simulink model "CoETS_TrqCalc"  (R2018a)
settings: configuration reference "cs_ert" (kept outside this file)
values from neighbouring files (symbols this model uses):
  DCSOVRDSENGPRT_SY : value not decoded    [CoETS_TrqCalc.sldd]
  ENGPRT_OVRDS_DCS : value not decoded    [CoETS_TrqCalc.sldd]
  PTPRTOVRDSSPDGOV_SY : value not decoded    [CoETS_TrqCalc.sldd]
  SPDGOV_OVRDS_PTPRT : value not decoded    [CoETS_TrqCalc.sldd]
settings Model: DataDictionary=CoETS_TrqCalc.sldd  Creator=zhoutinglin  LastModifiedBy=zhoutinglin

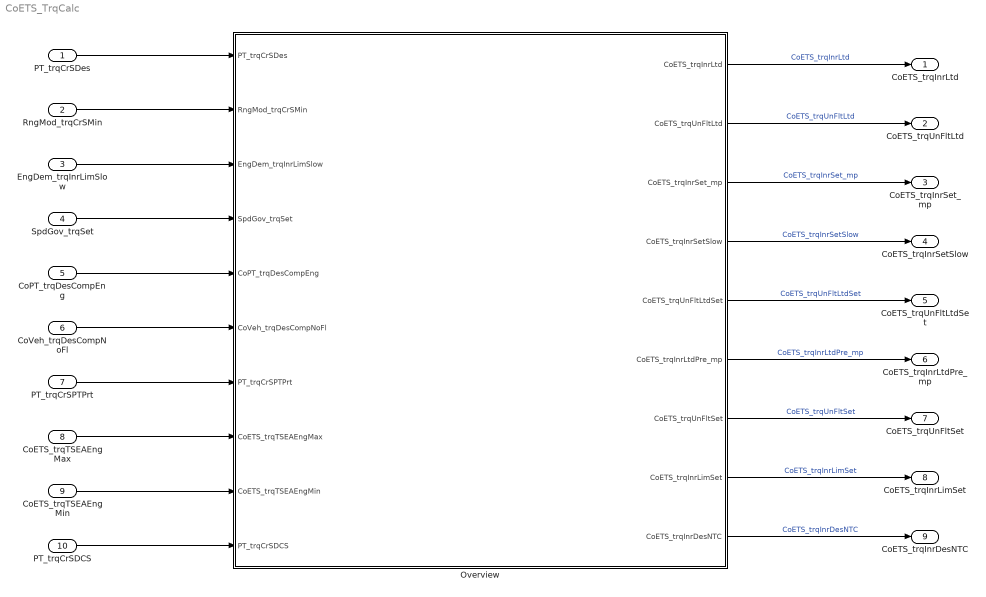
== system CoETS_TrqCalc ==
  PT_trqCrSDes : Inport  Description=application parameter for lead torque order to engine for rail pressure control（crankshaft torque）  OutMin=-3000  OutMax=3000  OutDataTypeStr=Torq  Unit=Nm  PortDimensions=[1 1]
  RngMod_trqCrSMin : Inport  Description=filtered setpoint torque of SpdGov  Port=2  OutMin=-3276.8  OutMax=3276.7  OutDataTypeStr=Torq  Unit=Nm  PortDimensions=[1 1]
  EngDem_trqInrLimSlow : Inport  Description=status speed control SpdGov  Port=3  OutMin=-3276.8  OutMax=3276.7  OutDataTypeStr=Torq  PortDimensions=[1 1]
  SpdGov_trqSet : Inport  Description=Resulting limiting torque (inner engine torque)  Port=4  OutMin=-3000  OutMax=3000  OutDataTypeStr=Torq  Unit=Nm  PortDimensions=[1 1]
  CoPT_trqDesCompEng : Inport  Description=inner engine limted lead torque  Port=5  OutMin=-3276  OutMax=3276  OutDataTypeStr=Torq  Unit=Nm  PortDimensions=[1 1]
  CoVeh_trqDesCompNoFl : Inport  Description=lead torque of SpdGov on the air path  Port=6  OutMin=-3000  OutMax=3000  OutDataTypeStr=Torq  Unit=Nm  PortDimensions=[1 1]
  PT_trqCrSPTPrt : Inport  Description=application parameter for lead torque order to engine（crankshaft torque）  Port=7  OutMin=-3000  OutMax=3000  OutDataTypeStr=Torq  Unit=Nm  PortDimensions=[1 1]
  CoETS_trqTSEAEngMax : Inport  Description=Application parameter for requested propulsion torque to engine(crankshaft torque)  Port=8  OutMin=-3276  OutMax=3276  OutDataTypeStr=Torq  Unit=Nm  PortDimensions=[1 1]
  CoETS_trqTSEAEngMin : Inport  Description=minimal crankshaft torque  Port=9  OutMin=-3276  OutMax=3276  OutDataTypeStr=Torq  Unit=Nm  PortDimensions=[1 1]
  PT_trqCrSDCS : Inport  Description=inner engine limted torque for Slow Path  Port=10  OutMin=-3000  OutMax=3000  OutDataTypeStr=Torq  Unit=Nm  PortDimensions=[1 1]
  Overview : Subsystem
  CoETS_trqInrLtd : Outport
  CoETS_trqUnFltLtd : Outport  Port=2
  CoETS_trqInrSet_mp : Outport  Port=3
  CoETS_trqInrSetSlow : Outport  Port=4
  CoETS_trqUnFltLtdSet : Outport  Port=5
  CoETS_trqInrLtdPre_mp : Outport  Port=6
  CoETS_trqUnFltSet : Outport  Port=7
  CoETS_trqInrLimSet : Outport  Port=8
  CoETS_trqInrDesNTC : Outport  Port=9
  wires:
  PT_trqCrSDes/1 -> Overview/1(PT_trqCrSDes)
  RngMod_trqCrSMin/1 -> Overview/2(RngMod_trqCrSMin)
  EngDem_trqInrLimSlow/1 -> Overview/3(EngDem_trqInrLimSlow)
  SpdGov_trqSet/1 -> Overview/4(SpdGov_trqSet)
  CoPT_trqDesCompEng/1 -> Overview/5(CoPT_trqDesCompEng)
  CoVeh_trqDesCompNoFl/1 -> Overview/6(CoVeh_trqDesCompNoFl)
  PT_trqCrSPTPrt/1 -> Overview/7(PT_trqCrSPTPrt)
  CoETS_trqTSEAEngMax/1 -> Overview/8(CoETS_trqTSEAEngMax)
  CoETS_trqTSEAEngMin/1 -> Overview/9(CoETS_trqTSEAEngMin)
  PT_trqCrSDCS/1 -> Overview/10(PT_trqCrSDCS)
  Overview/1(CoETS_trqInrLtd) -> CoETS_trqInrLtd/1  "CoETS_trqInrLtd"
  Overview/2(CoETS_trqUnFltLtd) -> CoETS_trqUnFltLtd/1  "CoETS_trqUnFltLtd"
  Overview/3(CoETS_trqInrSet_mp) -> CoETS_trqInrSet_mp/1  "CoETS_trqInrSet_mp"
  Overview/4(CoETS_trqInrSetSlow) -> CoETS_trqInrSetSlow/1  "CoETS_trqInrSetSlow"
  Overview/5(CoETS_trqUnFltLtdSet) -> CoETS_trqUnFltLtdSet/1  "CoETS_trqUnFltLtdSet"
  Overview/6(CoETS_trqInrLtdPre_mp) -> CoETS_trqInrLtdPre_mp/1  "CoETS_trqInrLtdPre_mp"
  Overview/7(CoETS_trqUnFltSet) -> CoETS_trqUnFltSet/1  "CoETS_trqUnFltSet"
  Overview/8(CoETS_trqInrLimSet) -> CoETS_trqInrLimSet/1  "CoETS_trqInrLimSet"
  Overview/9(CoETS_trqInrDesNTC) -> CoETS_trqInrDesNTC/1  "CoETS_trqInrDesNTC"

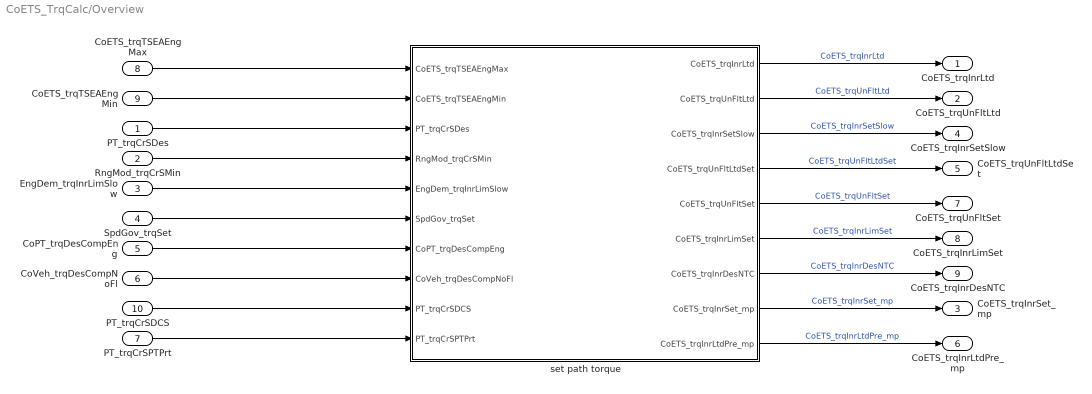
== system CoETS_TrqCalc/Overview ==
  PT_trqCrSDes : Inport  Tag=Nm  Description=Application parameter for requested propulsion torque to engine(crankshaft torque)  OutMin=-3000  OutMax=3000
  RngMod_trqCrSMin : Inport  Tag=Nm  Description=minimal crankshaft torque  Port=2  OutMin=-3276.8  OutMax=3276.7
  EngDem_trqInrLimSlow : Inport  Tag=Nm  Description=inner engine limted torque for Slow Path  Port=3  OutMin=-3276.8  OutMax=3276.7
  SpdGov_trqSet : Inport  Tag=Nm  Description=Set point torque of SpdGov on the fuel path  Port=4  OutMin=-3000  OutMax=3000
  CoPT_trqDesCompEng : Inport  Tag=Nm  Description=Application parameter for engine torque desired for compensation  Port=5  OutMin=-3276  OutMax=3276
  CoVeh_trqDesCompNoFl : Inport  Tag=Nm  Description=compensation torque with the shares,which not slur by the drive behaviour filter  Port=6  OutMin=-3000  OutMax=3000
  PT_trqCrSPTPrt : Inport  Tag=Nm  Description=Application parameter for powertrain protection train protection torque(crankshaft torque)  Port=7  OutMin=-3000  OutMax=3000
  CoETS_trqTSEAEngMax : Inport  Tag=Nm  Description=torque request to engine intervention decrement(Max)  Port=8  OutMin=-3276  OutMax=3276
  CoETS_trqTSEAEngMin : Inport  Tag=Nm  Description=torque request to engine intervention increment(Min)  Port=9  OutMin=-3276  OutMax=3276
  PT_trqCrSDCS : Inport  Tag=Nm  Description=crankshaft torque for request decrcment  Port=10  OutMin=-3000  OutMax=3000
  set path torque : Subsystem
  CoETS_trqInrLtd : Outport  Tag=Nm  Description=inner torque set value after limitation, before AS  OutMin=-3000  OutMax=3000
  CoETS_trqUnFltLtd : Outport  Tag=Nm  Description=Limited idle speed governor torque  Port=2  OutMin=-3276  OutMax=3276
  CoETS_trqInrSet_mp : Outport  Tag=Nm  Description=Intermediate inner torque for the set path without filteration  Port=3  OutMin=-3276  OutMax=3276
  CoETS_trqInrSetSlow : Outport  Tag=Nm  Description=Filtered inner torque ( positive torque) desired value (standard signal path) generated out of CoPT_trqDesEng  Port=4  OutMin=-3276  OutMax=3276
  CoETS_trqUnFltLtdSet : Outport  Tag=Nm  Description=Compensation torque of the accessories  Port=5  OutMin=-3276  OutMax=3276
  CoETS_trqInrLtdPre_mp : Outport  Tag=Nm  Description=inner set torque after limitation, before active surge damper  Port=6  OutMin=-3276  OutMax=3276
  CoETS_trqUnFltSet : Outport  Tag=Nm  Description="Compensation torque of \"loss torque compensation\" to bypass filter influences on the set path which is partly compensated"  Port=7  OutMin=-3276  OutMax=3276
  CoETS_trqInrLimSet : Outport  Tag=Nm  Description=Limitation torque without the part of the speed governor  Port=8  OutMin=-3000  OutMax=3000
  CoETS_trqInrDesNTC : Outport  Tag=Nm  Description=Additional desired engine friction Nm  Port=9  OutMin=-3276  OutMax=3276
  wires:
  set path torque/2(CoETS_trqUnFltLtd) -> CoETS_trqUnFltLtd/1  "CoETS_trqUnFltLtd"
  set path torque/4(CoETS_trqUnFltLtdSet) -> CoETS_trqUnFltLtdSet/1  "CoETS_trqUnFltLtdSet"
  SpdGov_trqSet/1 -> set path torque/6(SpdGov_trqSet)
  set path torque/7(CoETS_trqInrDesNTC) -> CoETS_trqInrDesNTC/1  "CoETS_trqInrDesNTC"
  set path torque/6(CoETS_trqInrLimSet) -> CoETS_trqInrLimSet/1  "CoETS_trqInrLimSet"
  CoVeh_trqDesCompNoFl/1 -> set path torque/8(CoVeh_trqDesCompNoFl)
  RngMod_trqCrSMin/1 -> set path torque/4(RngMod_trqCrSMin)
  set path torque/1(CoETS_trqInrLtd) -> CoETS_trqInrLtd/1  "CoETS_trqInrLtd"
  CoPT_trqDesCompEng/1 -> set path torque/7(CoPT_trqDesCompEng)
  set path torque/8(CoETS_trqInrSet_mp) -> CoETS_trqInrSet_mp/1  "CoETS_trqInrSet_mp"
  set path torque/9(CoETS_trqInrLtdPre_mp) -> CoETS_trqInrLtdPre_mp/1  "CoETS_trqInrLtdPre_mp"
  PT_trqCrSPTPrt/1 -> set path torque/10(PT_trqCrSPTPrt)
  set path torque/3(CoETS_trqInrSetSlow) -> CoETS_trqInrSetSlow/1  "CoETS_trqInrSetSlow"
  CoETS_trqTSEAEngMax/1 -> set path torque/1(CoETS_trqTSEAEngMax)
  PT_trqCrSDes/1 -> set path torque/3(PT_trqCrSDes)
  set path torque/5(CoETS_trqUnFltSet) -> CoETS_trqUnFltSet/1  "CoETS_trqUnFltSet"
  PT_trqCrSDCS/1 -> set path torque/9(PT_trqCrSDCS)
  EngDem_trqInrLimSlow/1 -> set path torque/5(EngDem_trqInrLimSlow)
  CoETS_trqTSEAEngMin/1 -> set path torque/2(CoETS_trqTSEAEngMin)

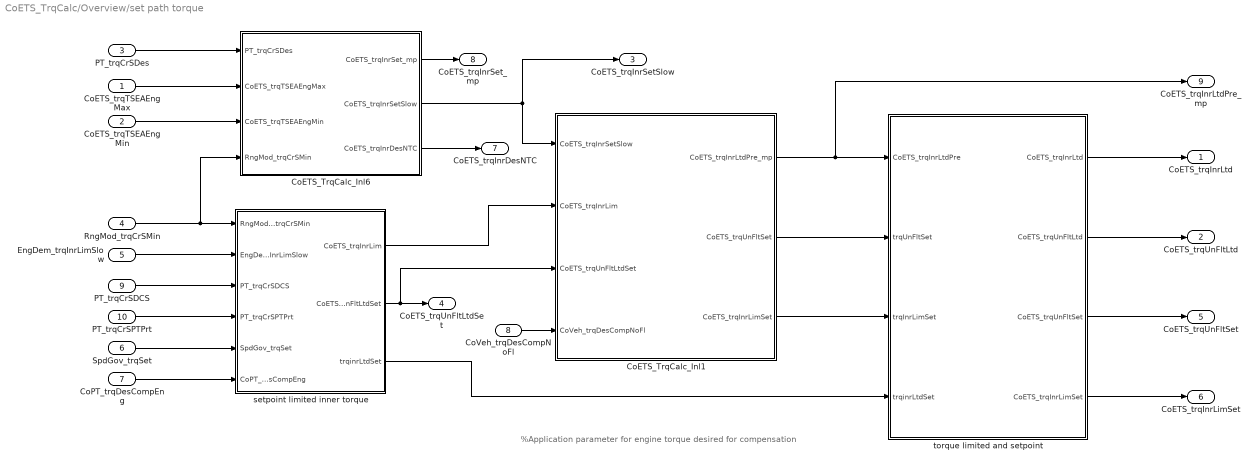
== system CoETS_TrqCalc/Overview/set path torque ==
  note: %Application parameter for engine torque desired for compensation
  CoETS_trqTSEAEngMax : Inport
  CoETS_trqTSEAEngMin : Inport  Port=2
  PT_trqCrSDes : Inport  Port=3
  RngMod_trqCrSMin : Inport  Port=4
  EngDem_trqInrLimSlow : Inport  Port=5
  SpdGov_trqSet : Inport  Port=6
  CoPT_trqDesCompEng : Inport  Port=7
  CoVeh_trqDesCompNoFl : Inport  Port=8
  PT_trqCrSDCS : Inport  Port=9
  PT_trqCrSPTPrt : Inport  Port=10
  CoETS_TrqCalc_Inl1 : Subsystem
  CoETS_TrqCalc_Inl6 : Subsystem
  setpoint limited inner torque : Subsystem
  torque limited and setpoint : Subsystem
  CoETS_trqInrLtd : Outport
  CoETS_trqUnFltLtd : Outport  Port=2
  CoETS_trqInrSetSlow : Outport  Port=3
  CoETS_trqUnFltLtdSet : Outport  Port=4
  CoETS_trqUnFltSet : Outport  Port=5
  CoETS_trqInrLimSet : Outport  Port=6
  CoETS_trqInrDesNTC : Outport  Port=7
  CoETS_trqInrSet_mp : Outport  Port=8
  CoETS_trqInrLtdPre_mp : Outport  Port=9
  wires:
  RngMod_trqCrSMin/1 -> CoETS_TrqCalc_Inl6/4(RngMod_trqCrSMin), setpoint limited inner torque/1(RngMod_trqCrSMin)
  PT_trqCrSDes/1 -> CoETS_TrqCalc_Inl6/1(PT_trqCrSDes)
  CoETS_trqTSEAEngMax/1 -> CoETS_TrqCalc_Inl6/2(CoETS_trqTSEAEngMax)
  CoETS_trqTSEAEngMin/1 -> CoETS_TrqCalc_Inl6/3(CoETS_trqTSEAEngMin)
  CoVeh_trqDesCompNoFl/1 -> CoETS_TrqCalc_Inl1/4(CoVeh_trqDesCompNoFl)
  setpoint limited inner torque/2(CoETS_trqUnFltLtdSet) -> CoETS_trqUnFltLtdSet/1, CoETS_TrqCalc_Inl1/3(CoETS_trqUnFltLtdSet)
  EngDem_trqInrLimSlow/1 -> setpoint limited inner torque/2(EngDem_trqInrLimSlow)
  PT_trqCrSDCS/1 -> setpoint limited inner torque/3(PT_trqCrSDCS)
  PT_trqCrSPTPrt/1 -> setpoint limited inner torque/4(PT_trqCrSPTPrt)
  SpdGov_trqSet/1 -> setpoint limited inner torque/5(SpdGov_trqSet)
  CoPT_trqDesCompEng/1 -> setpoint limited inner torque/6(CoPT_trqDesCompEng)
  setpoint limited inner torque/1(CoETS_trqInrLim) -> CoETS_TrqCalc_Inl1/2(CoETS_trqInrLim)
  CoETS_TrqCalc_Inl6/1(CoETS_trqInrSet_mp) -> CoETS_trqInrSet_mp/1
  CoETS_TrqCalc_Inl6/2(CoETS_trqInrSetSlow) -> CoETS_trqInrSetSlow/1, CoETS_TrqCalc_Inl1/1(CoETS_trqInrSetSlow)
  CoETS_TrqCalc_Inl6/3(CoETS_trqInrDesNTC) -> CoETS_trqInrDesNTC/1
  CoETS_TrqCalc_Inl1/1(CoETS_trqInrLtdPre_mp) -> CoETS_trqInrLtdPre_mp/1, torque limited and setpoint/1(CoETS_trqInrLtdPre)
  CoETS_TrqCalc_Inl1/2(CoETS_trqUnFltSet) -> torque limited and setpoint/2(trqUnFltSet)
  CoETS_TrqCalc_Inl1/3(CoETS_trqInrLimSet) -> torque limited and setpoint/3(trqInrLimSet)
  setpoint limited inner torque/3(trqinrLtdSet) -> torque limited and setpoint/4(trqinrLtdSet)
  torque limited and setpoint/1(CoETS_trqInrLtd) -> CoETS_trqInrLtd/1
  torque limited and setpoint/2(CoETS_trqUnFltLtd) -> CoETS_trqUnFltLtd/1
  torque limited and setpoint/3(CoETS_trqUnFltSet) -> CoETS_trqUnFltSet/1
  torque limited and setpoint/4(CoETS_trqInrLimSet) -> CoETS_trqInrLimSet/1

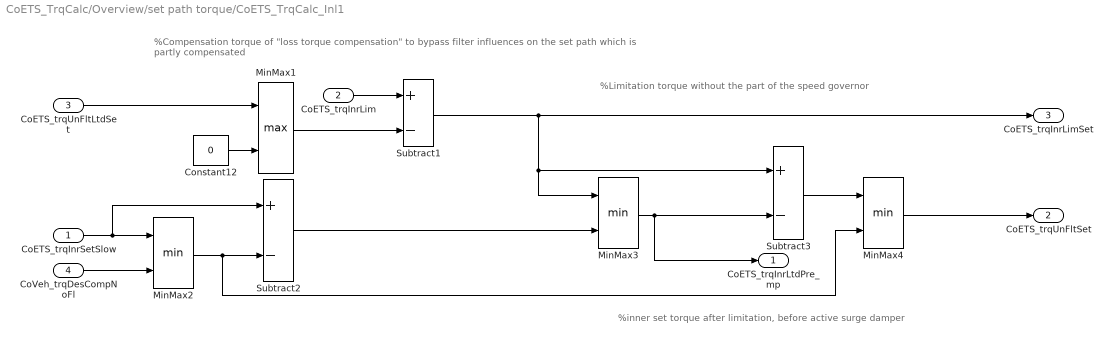
== system CoETS_TrqCalc/Overview/set path torque/CoETS_TrqCalc_Inl1 ==
  note: %Limitation torque without the part of the speed governor
  note: %inner set torque after limitation, before active surge damper
  note: %Compensation torque of "loss torque compensation" to bypass filter influences on the set path which is partly compensated
  CoETS_trqInrSetSlow : Inport
  CoETS_trqInrLim : Inport  Port=2
  CoETS_trqUnFltLtdSet : Inport  Port=3
  CoVeh_trqDesCompNoFl : Inport  Port=4
  Constant12 : Constant  Value=0  VectorParams1D=off  OutDataTypeStr=Inherit: Inherit via back propagation
  MinMax1 : MinMax  Function=max  Inputs=2  InputSameDT=on
  MinMax2 : MinMax  Inputs=2  InputSameDT=on
  MinMax3 : MinMax  Inputs=2  InputSameDT=on
  MinMax4 : MinMax  Inputs=2  InputSameDT=on
  Subtract1 : Sum  Inputs=+-  OutDataTypeStr=Inherit: Inherit via back propagation  SaturateOnIntegerOverflow=on  InputSameDT=on
  Subtract2 : Sum  Inputs=+-  OutDataTypeStr=Inherit: Inherit via back propagation  SaturateOnIntegerOverflow=on  InputSameDT=on
  Subtract3 : Sum  Inputs=+-  OutDataTypeStr=Inherit: Inherit via back propagation  SaturateOnIntegerOverflow=on  InputSameDT=on
  CoETS_trqInrLtdPre_mp : Outport
  CoETS_trqUnFltSet : Outport  Port=2
  CoETS_trqInrLimSet : Outport  Port=3
  wires:
  MinMax4/1 -> CoETS_trqUnFltSet/1
  Subtract3/1 -> MinMax4/1
  MinMax3/1 -> CoETS_trqInrLtdPre_mp/1, Subtract3/2
  Subtract1/1 -> CoETS_trqInrLimSet/1, Subtract3/1, MinMax3/1
  Subtract2/1 -> MinMax3/2
  MinMax2/1 -> Subtract2/2, MinMax4/2
  CoVeh_trqDesCompNoFl/1 -> MinMax2/2
  CoETS_trqInrSetSlow/1 -> MinMax2/1, Subtract2/1
  MinMax1/1 -> Subtract1/2
  CoETS_trqUnFltLtdSet/1 -> MinMax1/1
  Constant12/1 -> MinMax1/2
  CoETS_trqInrLim/1 -> Subtract1/1

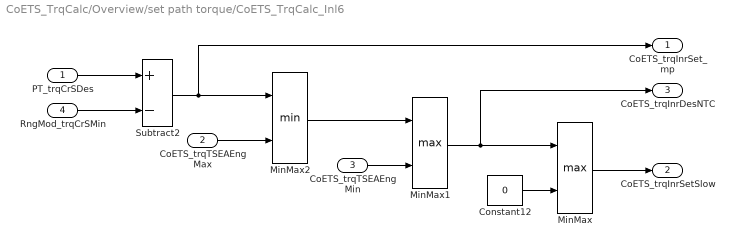
== system CoETS_TrqCalc/Overview/set path torque/CoETS_TrqCalc_Inl6 ==
  PT_trqCrSDes : Inport
  CoETS_trqTSEAEngMax : Inport  Port=2
  CoETS_trqTSEAEngMin : Inport  Port=3
  RngMod_trqCrSMin : Inport  Port=4
  Constant12 : Constant  Value=0  VectorParams1D=off  OutDataTypeStr=Inherit: Inherit via back propagation
  MinMax : MinMax  Function=max  Inputs=2  InputSameDT=on
  MinMax1 : MinMax  Function=max  Inputs=2  InputSameDT=on
  MinMax2 : MinMax  Inputs=2  InputSameDT=on
  Subtract2 : Sum  Inputs=+-  OutDataTypeStr=Inherit: Inherit via back propagation  SaturateOnIntegerOverflow=on  InputSameDT=on
  CoETS_trqInrSet_mp : Outport
  CoETS_trqInrSetSlow : Outport  Port=2
  CoETS_trqInrDesNTC : Outport  Port=3
  wires:
  CoETS_trqTSEAEngMin/1 -> MinMax1/2
  RngMod_trqCrSMin/1 -> Subtract2/2
  PT_trqCrSDes/1 -> Subtract2/1
  Subtract2/1 -> MinMax2/1, CoETS_trqInrSet_mp/1
  MinMax/1 -> CoETS_trqInrSetSlow/1
  Constant12/1 -> MinMax/2
  MinMax1/1 -> MinMax/1, CoETS_trqInrDesNTC/1
  CoETS_trqTSEAEngMax/1 -> MinMax2/2
  MinMax2/1 -> MinMax1/1

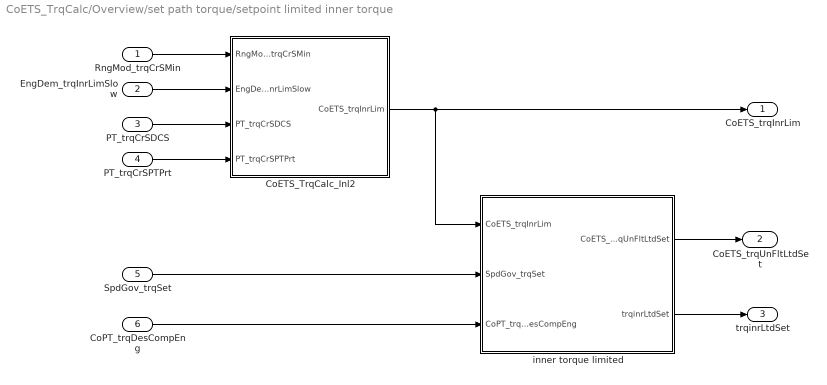
== system CoETS_TrqCalc/Overview/set path torque/setpoint limited inner torque ==
  RngMod_trqCrSMin : Inport
  EngDem_trqInrLimSlow : Inport  Port=2
  PT_trqCrSDCS : Inport  Port=3
  PT_trqCrSPTPrt : Inport  Port=4
  SpdGov_trqSet : Inport  Port=5
  CoPT_trqDesCompEng : Inport  Port=6
  CoETS_TrqCalc_Inl2 : Subsystem
  inner torque limited : Subsystem
  CoETS_trqInrLim : Outport
  CoETS_trqUnFltLtdSet : Outport  Port=2
  trqinrLtdSet : Outport  Port=3
  wires:
  EngDem_trqInrLimSlow/1 -> CoETS_TrqCalc_Inl2/2(EngDem_trqInrLimSlow)
  PT_trqCrSPTPrt/1 -> CoETS_TrqCalc_Inl2/4(PT_trqCrSPTPrt)
  PT_trqCrSDCS/1 -> CoETS_TrqCalc_Inl2/3(PT_trqCrSDCS)
  RngMod_trqCrSMin/1 -> CoETS_TrqCalc_Inl2/1(RngMod_trqCrSMin)
  SpdGov_trqSet/1 -> inner torque limited/2(SpdGov_trqSet)
  CoPT_trqDesCompEng/1 -> inner torque limited/3(CoPT_trqDesCompEng)
  inner torque limited/1(CoETS_trqUnFltLtdSet) -> CoETS_trqUnFltLtdSet/1
  inner torque limited/2(trqinrLtdSet) -> trqinrLtdSet/1
  CoETS_TrqCalc_Inl2/1(CoETS_trqInrLim) -> inner torque limited/1(CoETS_trqInrLim), CoETS_trqInrLim/1

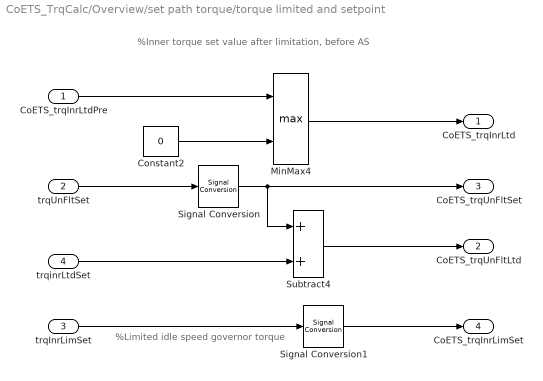
== system CoETS_TrqCalc/Overview/set path torque/torque limited and setpoint ==
  note: %Inner torque set value after limitation, before AS
  note: %Limited idle speed governor torque
  CoETS_trqInrLtdPre : Inport
  trqUnFltSet : Inport  Port=2
  trqInrLimSet : Inport  Port=3
  trqinrLtdSet : Inport  Port=4
  Constant2 : Constant  Value=0  VectorParams1D=off  OutDataTypeStr=Inherit: Inherit via back propagation
  MinMax4 : MinMax  Function=max  Inputs=2  InputSameDT=on
  Signal Conversion : SignalConversion  OverrideOpt=off
  Signal Conversion1 : SignalConversion  OverrideOpt=off
  Subtract4 : Sum  OutDataTypeStr=Inherit: Inherit via back propagation  SaturateOnIntegerOverflow=on  InputSameDT=on
  CoETS_trqInrLtd : Outport
  CoETS_trqUnFltLtd : Outport  Port=2
  CoETS_trqUnFltSet : Outport  Port=3
  CoETS_trqInrLimSet : Outport  Port=4
  wires:
  CoETS_trqInrLtdPre/1 -> MinMax4/1
  MinMax4/1 -> CoETS_trqInrLtd/1
  trqUnFltSet/1 -> Signal Conversion/1
  Constant2/1 -> MinMax4/2
  trqInrLimSet/1 -> Signal Conversion1/1
  Subtract4/1 -> CoETS_trqUnFltLtd/1
  trqinrLtdSet/1 -> Subtract4/2
  Signal Conversion/1 -> Subtract4/1, CoETS_trqUnFltSet/1
  Signal Conversion1/1 -> CoETS_trqInrLimSet/1

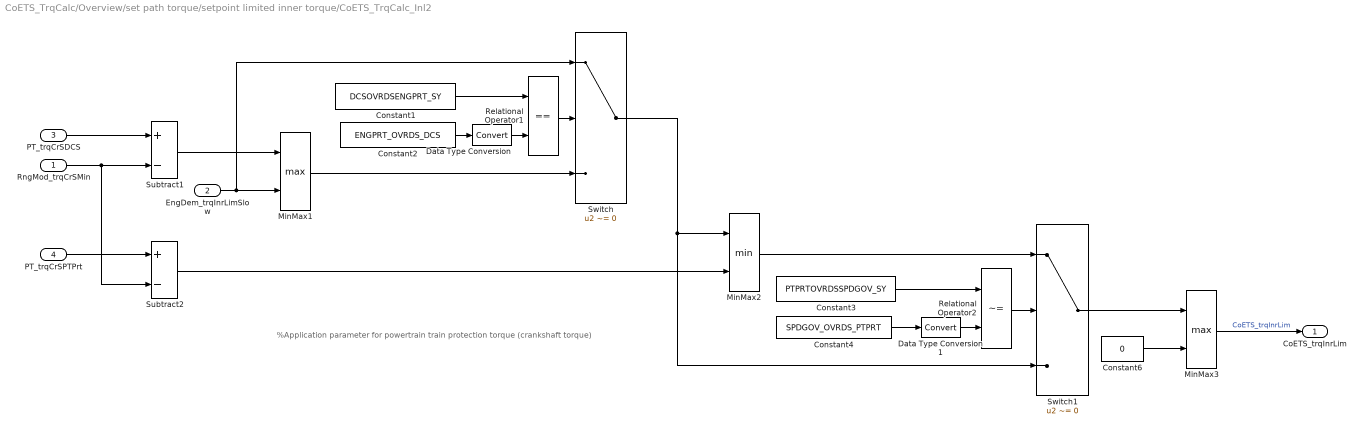
== system CoETS_TrqCalc/Overview/set path torque/setpoint limited inner torque/CoETS_TrqCalc_Inl2 ==
  note: %Application parameter for powertrain train protection torque (crankshaft torque)
  RngMod_trqCrSMin : Inport
  EngDem_trqInrLimSlow : Inport  Port=2
  PT_trqCrSDCS : Inport  Port=3
  PT_trqCrSPTPrt : Inport  Port=4
  Constant1 : Constant  Value=DCSOVRDSENGPRT_SY  VectorParams1D=off
  Constant2 : Constant  Value=ENGPRT_OVRDS_DCS  VectorParams1D=off
  Constant3 : Constant  Value=PTPRTOVRDSSPDGOV_SY  VectorParams1D=off
  Constant4 : Constant  Value=SPDGOV_OVRDS_PTPRT  VectorParams1D=off
  Constant6 : Constant  Value=0  VectorParams1D=off  OutDataTypeStr=Inherit: Inherit via back propagation
  Data Type Conversion : DataTypeConversion
  Data Type Conversion1 : DataTypeConversion
  MinMax1 : MinMax  Function=max  Inputs=2  InputSameDT=on
  MinMax2 : MinMax  Inputs=2  InputSameDT=on
  MinMax3 : MinMax  Function=max  Inputs=2  InputSameDT=on
  Relational Operator1 : RelationalOperator  Operator===  OutDataTypeStr=boolean  RndMeth=Simplest  InputSameDT=on
  Relational Operator2 : RelationalOperator  Operator=~=  OutDataTypeStr=boolean  RndMeth=Simplest  InputSameDT=on
  Subtract1 : Sum  Inputs=+-  OutDataTypeStr=Inherit: Inherit via back propagation  SaturateOnIntegerOverflow=on  InputSameDT=on
  Subtract2 : Sum  Inputs=+-  OutDataTypeStr=Inherit: Inherit via back propagation  SaturateOnIntegerOverflow=on  InputSameDT=on
  Switch : Switch  Criteria=u2 ~= 0  OutDataTypeStr=Inherit: Inherit via back propagation  SaturateOnIntegerOverflow=on  InputSameDT=on
  Switch1 : Switch  Criteria=u2 ~= 0  OutDataTypeStr=Inherit: Inherit via back propagation  SaturateOnIntegerOverflow=on  InputSameDT=on
  CoETS_trqInrLim : Outport
  wires:
  Data Type Conversion1/1 -> Relational Operator2/2
  Data Type Conversion/1 -> Relational Operator1/2
  MinMax3/1 -> CoETS_trqInrLim/1  "CoETS_trqInrLim"
  Constant6/1 -> MinMax3/2
  Switch1/1 -> MinMax3/1
  Relational Operator2/1 -> Switch1/2
  MinMax2/1 -> Switch1/1
  Switch/1 -> Switch1/3, MinMax2/1
  Subtract2/1 -> MinMax2/2
  RngMod_trqCrSMin/1 -> Subtract1/2, Subtract2/2
  PT_trqCrSPTPrt/1 -> Subtract2/1
  Relational Operator1/1 -> Switch/2
  MinMax1/1 -> Switch/3
  EngDem_trqInrLimSlow/1 -> MinMax1/2, Switch/1
  Subtract1/1 -> MinMax1/1
  PT_trqCrSDCS/1 -> Subtract1/1
  Constant4/1 -> Data Type Conversion1/1
  Constant3/1 -> Relational Operator2/1
  Constant2/1 -> Data Type Conversion/1
  Constant1/1 -> Relational Operator1/1

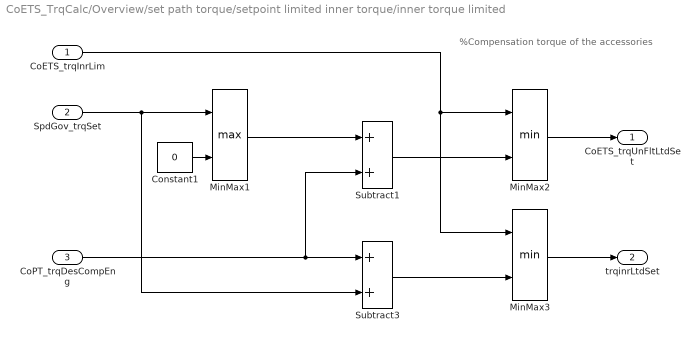
== system CoETS_TrqCalc/Overview/set path torque/setpoint limited inner torque/inner torque limited ==
  note: %Compensation torque of the accessories
  CoETS_trqInrLim : Inport
  SpdGov_trqSet : Inport  Port=2
  CoPT_trqDesCompEng : Inport  Port=3
  Constant1 : Constant  Value=0  VectorParams1D=off  OutDataTypeStr=Inherit: Inherit via back propagation
  MinMax1 : MinMax  Function=max  Inputs=2  InputSameDT=on
  MinMax2 : MinMax  Inputs=2  InputSameDT=on
  MinMax3 : MinMax  Inputs=2  InputSameDT=on
  Subtract1 : Sum  OutDataTypeStr=Inherit: Inherit via back propagation  SaturateOnIntegerOverflow=on  InputSameDT=on
  Subtract3 : Sum  OutDataTypeStr=Inherit: Inherit via back propagation  SaturateOnIntegerOverflow=on  InputSameDT=on
  CoETS_trqUnFltLtdSet : Outport
  trqinrLtdSet : Outport  Port=2
  wires:
  MinMax1/1 -> Subtract1/1
  MinMax3/1 -> trqinrLtdSet/1
  Subtract3/1 -> MinMax3/2
  Subtract1/1 -> MinMax2/2
  CoPT_trqDesCompEng/1 -> Subtract1/2, Subtract3/1
  Constant1/1 -> MinMax1/2
  SpdGov_trqSet/1 -> MinMax1/1, Subtract3/2
  MinMax2/1 -> CoETS_trqUnFltLtdSet/1
  CoETS_trqInrLim/1 -> MinMax3/1, MinMax2/1
